simulink model "ch_11_p_19"  (R2022b)
settings: Solver=VariableStepAuto  StartTime=0.0  StopTime=1  RelTol=1e-3
settings Model: Creator=Mahadevu Sudheer  LastModifiedBy=Mahadevu Sudheer

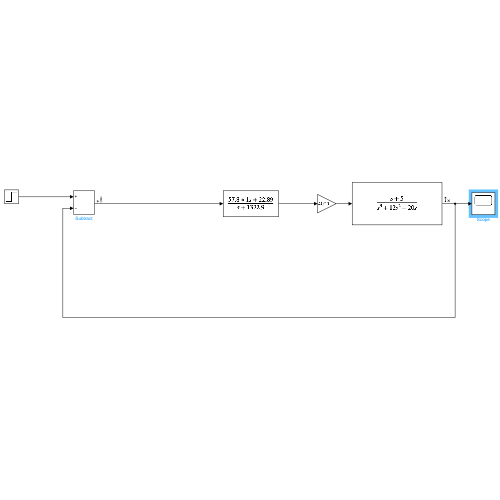
[thumbnail: Simulink's stored preview of the top-level diagram]
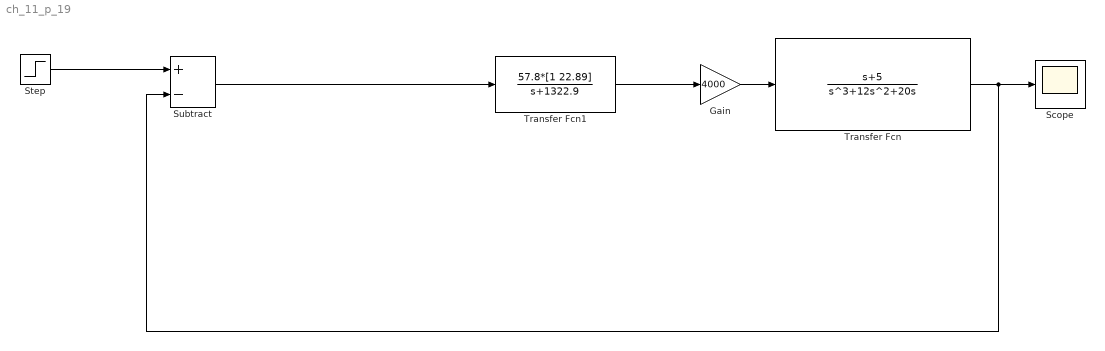
== system ch_11_p_19 ==
  Gain : Gain  Gain=4000
  Scope : Scope
  Step : Step  Time=0  SampleTime=0
  Subtract : Sum  Inputs=+-
  Transfer Fcn : TransferFcn  Numerator=[1 5]  Denominator=[1 12 20 0]
  Transfer Fcn1 : TransferFcn  Numerator=57.8*[1 22.89]  Denominator=[1 1322.9]
  wires:
  Gain/1 -> Transfer Fcn/1
  Subtract/1 -> Transfer Fcn1/1
  Step/1 -> Subtract/1
  Transfer Fcn/1 -> Subtract/2, Scope/1
  Transfer Fcn1/1 -> Gain/1
